simulink model "SF003A_Dampg"  (R2013b)
settings: Solver=FixedStepDiscrete  SolverMode=SingleTasking  StartTime=0.0  StopTime=1  FixedStep=.002  RelTol=1e-3
values from neighbouring files (symbols this model uses):
  ARCHGLBPRM_2MILLISEC_SEC_F32 = DataDict.Constant    [SF003A_Dampg_DataDict.m]
  DampgHydBasCoeff1 = DataDict.Calibration    [SF003A_Dampg_DataDict.m]
  DampgHydBasCoeff2 = DataDict.Calibration    [SF003A_Dampg_DataDict.m]
  DampgHydBasCoeff3 = DataDict.Calibration    [SF003A_Dampg_DataDict.m]
  DampgHydBasCoeff4 = DataDict.Calibration    [SF003A_Dampg_DataDict.m]
  DampgHydOutpLim = DataDict.Calibration    [SF003A_Dampg_DataDict.m]
  DampgQuad13Mplr = DataDict.Calibration    [SF003A_Dampg_DataDict.m]
  DampgQuad24Mplr = DataDict.Calibration    [SF003A_Dampg_DataDict.m]
  DampgQuadHwTqBacklsh = DataDict.Calibration    [SF003A_Dampg_DataDict.m]
  DampgQuadMotVelBacklsh = DataDict.Calibration    [SF003A_Dampg_DataDict.m]
  FLTINJ_DAMPG_DAMPGCMDBAS = DataDict.Constant    [SF003A_Dampg_DataDict.m]
libraries: FloatToFixd x9, Fil x8, FixdToFloat x8, LnrIntrpn x7, NxtrAbslt x5, NxtrSign x3, NxtrLim x3, simulink x1, NxtrMax x1, BilnrIntrpnMplX x1
(part 2 of 2)

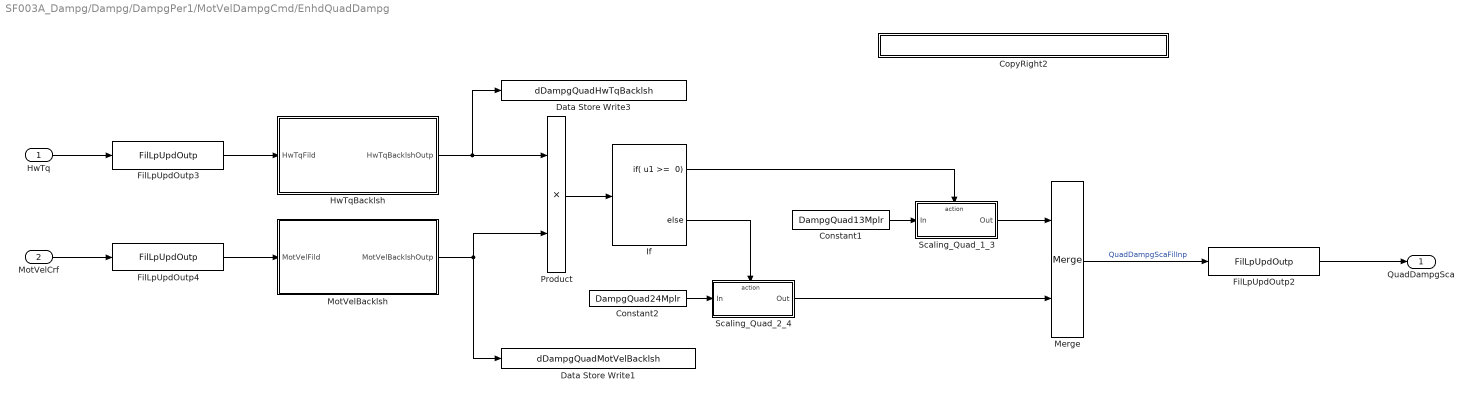
== system SF003A_Dampg/Dampg/DampgPer1/MotVelDampgCmd/EnhdQuadDampg  ==
  HwTq : Inport
  MotVelCrf : Inport  Port=2
  Constant1 : Constant  RequirementInfo={'linktype_rmi_doors' '0000a525 (/E-STEER Core/SubSystem Specifications/Application Functions/SF003A Damping)' '#SF003A_113' 'true' 'REQ: SF003A_113' '' } %GIDa_5b902024_3e8c_4494_84c3_91dcbfea766a  Value=DampgQuad13Mplr  OutDataTypeStr=single
  Constant2 : Constant  RequirementInfo={'linktype_rmi_doors' '0000a525 (/E-STEER Core/SubSystem Specifications/Application Functions/SF003A Damping)' '#SF003A_114' 'true' 'REQ: SF003A_114' '' } %GIDa_587e475f_d2d7_438f_8480_63dc4e95efa6  Value=DampgQuad24Mplr  OutDataTypeStr=single
  CopyRight2 : Subsystem  Description=|  mask(Copyright Information){none=on}
      | Copyright info block.                                               
      |                                                                     
      | Place copyright information at the top of every subsystem in design.
      mask prompts: none "No parameters"
      mask help: Place copyright information at the top of every subsystem in design.
      mask Display:
      | NxtrConf = 'Nexteer Confidential';
      | 
      | sys = bdroot; %handle for the current model ("system")
      | first = get_param(sys,'Created');
      | if(isempty(first))
      |     first = datestr(now,'yyyy');
      | else
      |     first = first(end-3:end);  %year is last four digits
      | end
      | 
      | last = get_param(sys,'LastModifiedDate');
      | if isempty(last)
      |     last = datestr(now,'yyyy');
      | else
      |     last = last(end-3:end);
      | end
      | 
      | if strcmp(first,last)
      |     fprintf('%s -- Copyright %s Nexteer',NxtrConf,first)
      | else
      |     fprintf('%s -- %s%s- %s Nexteer',NxtrConf,char(169),first,last)
      | end
  Data Store Write1 : DataStoreWrite  DataStoreName=dDampgQuadMotVelBacklsh
  Data Store Write3 : DataStoreWrite  DataStoreName=dDampgQuadHwTqBacklsh
  FilLpUpdOutp2 : Fil/FilLpUpdOutp  RequirementInfo={'linktype_rmi_doors' '0000a525 (/E-STEER Core/SubSystem Specifications/Application Functions/SF003A Damping)' '#SF003A_115' 'true' 'REQ: SF003A_115' '' } %GIDa_3cce034f_6843_47ba_883e_e9472d6bea51  StVar=QuadDampgScaLpFil
      settings: AttributesFormatString=StVar: %<StVar>
  FilLpUpdOutp3 : Fil/FilLpUpdOutp  RequirementInfo={'linktype_rmi_doors' '0000a525 (/E-STEER Core/SubSystem Specifications/Application Functions/SF003A Damping)' '#SF003A_135' 'true' 'REQ: SF003A_135' '' } %GIDa_4951c7ec_0e7d_4afa_9064_51627a057340  StVar=QuadDampgHwTqLpFil
      settings: AttributesFormatString=StVar: %<StVar>
  FilLpUpdOutp4 : Fil/FilLpUpdOutp  RequirementInfo={'linktype_rmi_doors' '0000a525 (/E-STEER Core/SubSystem Specifications/Application Functions/SF003A Damping)' '#SF003A_137' 'true' 'REQ: SF003A_137' '' } %GIDa_73f2fc1e_0696_4bfb_b3f7_ed9952c3095a  StVar=QuadDampgMotVelLpFil
      settings: AttributesFormatString=StVar: %<StVar>
  HwTqBacklsh : Subsystem  RequirementInfo={'linktype_rmi_doors' '0000a525 (/E-STEER Core/SubSystem Specifications/Application Functions/SF003A Damping)' '#SF003A_136' 'true' 'REQ: SF003A_136' '' } %GIDa_bd470be9_d6d9_40e9_857a_c378f7458848
  If : If  RequirementInfo={'linktype_rmi_doors' '0000a525 (/E-STEER Core/SubSystem Specifications/Application Functions/SF003A Damping)' '#SF003A_113' 'true' 'REQ: SF003A_113' '' ; 'linktype_rmi_doors' '0000a525 (/E-STEER Core/SubSystem Specifications/Application Functions/SF003A Damping)' '#SF003A_114' 'true' 'REQ: SF003A_114' '' } %GIDa_cfe1943d_8645_4c6c_ae36_bf006afd8732  IfExpression="u1 >=  0"
  Merge : Merge
  MotVelBacklsh : Subsystem  RequirementInfo={'linktype_rmi_doors' '0000a525 (/E-STEER Core/SubSystem Specifications/Application Functions/SF003A Damping)' '#SF003A_138' 'true' 'REQ: SF003A_138' '' } %GIDa_e894bb2d_e794_4ed4_a57e_9441dd65fceb
  Product : Product  RndMeth=Zero
  Scaling_Quad_1_3 : Subsystem  RequirementInfo={'linktype_rmi_doors' '0000a525 (/E-STEER Core/SubSystem Specifications/Application Functions/SF003A Damping)' '#SF003A_113' 'true' 'REQ: SF003A_113' '' } %GIDa_485cad3f_31a8_4856_95a7_16cb3f5dc668  TreatAsAtomicUnit=on
  Scaling_Quad_2_4 : Subsystem  RequirementInfo={'linktype_rmi_doors' '0000a525 (/E-STEER Core/SubSystem Specifications/Application Functions/SF003A Damping)' '#SF003A_114' 'true' 'REQ: SF003A_114' '' } %GIDa_b28b5c6d_494b_445a_b5ee_da8ce8308b9a  TreatAsAtomicUnit=on
  QuadDampgSca : Outport
  wires:
  MotVelCrf/1 -> FilLpUpdOutp4/1
  HwTq/1 -> FilLpUpdOutp3/1
  MotVelBacklsh/1(MotVelBacklshOutp) -> Data Store Write1/1, Product/2
  Product/1 -> If/1
  If/1 -> Scaling_Quad_1_3/Action
  If/2 -> Scaling_Quad_2_4/Action
  Scaling_Quad_1_3/1(Out) -> Merge/1
  Merge/1 -> FilLpUpdOutp2/1  "QuadDampgScaFilInp"
  FilLpUpdOutp2/1 -> QuadDampgSca/1
  Constant1/1 -> Scaling_Quad_1_3/1(In)
  Constant2/1 -> Scaling_Quad_2_4/1(In)
  Scaling_Quad_2_4/1(Out) -> Merge/2
  FilLpUpdOutp4/1 -> MotVelBacklsh/1(MotVelFild)
  HwTqBacklsh/1(HwTqBacklshOutp) -> Data Store Write3/1, Product/1
  FilLpUpdOutp3/1 -> HwTqBacklsh/1(HwTqFild)

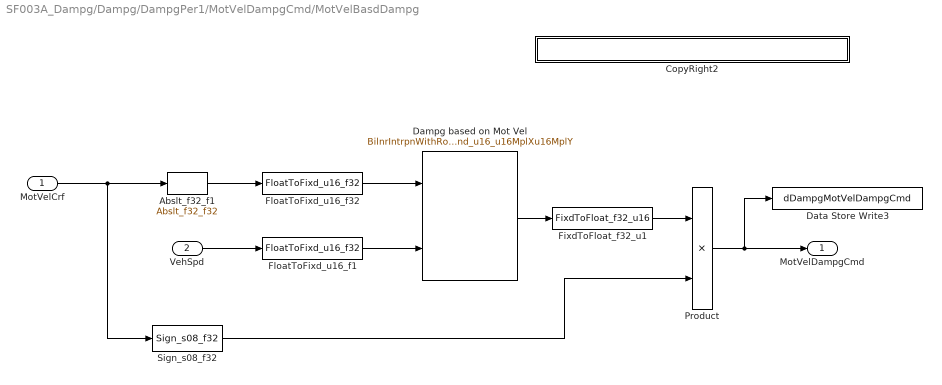
== system SF003A_Dampg/Dampg/DampgPer1/MotVelDampgCmd/MotVelBasdDampg ==
  MotVelCrf : Inport
  VehSpd : Inport  Port=2
  Abslt_f32_f1 : NxtrAbslt/Abslt_f32_f32  SFunctionSpec=single y1 = Abslt_f32_f32(single u1)
      settings: AttributesFormatString=%<Name>
  CopyRight2 : Subsystem  Description=|  mask(Copyright Information){none=on}
      | Copyright info block.                                               
      |                                                                     
      | Place copyright information at the top of every subsystem in design.
      mask prompts: none "No parameters"
      mask help: Place copyright information at the top of every subsystem in design.
      mask Display:
      | NxtrConf = 'Nexteer Confidential';
      | 
      | sys = bdroot; %handle for the current model ("system")
      | first = get_param(sys,'Created');
      | if(isempty(first))
      |     first = datestr(now,'yyyy');
      | else
      |     first = first(end-3:end);  %year is last four digits
      | end
      | 
      | last = get_param(sys,'LastModifiedDate');
      | if isempty(last)
      |     last = datestr(now,'yyyy');
      | else
      |     last = last(end-3:end);
      | end
      | 
      | if strcmp(first,last)
      |     fprintf('%s -- Copyright %s Nexteer',NxtrConf,first)
      | else
      |     fprintf('%s -- %s%s- %s Nexteer',NxtrConf,char(169),first,last)
      | end
  Dampg based on Mot Vel : BilnrIntrpnMplX/BilnrIntrpnWithRound_u16_u16MplXu16MplY  RequirementInfo={'linktype_rmi_doors' '0000a525 (/E-STEER Core/SubSystem Specifications/Application Functions/SF003A Damping)' '#SF003A_116' 'true' 'REQ: SF003A_116' '' } %GIDa_ea730993_70af_440c_875a_3fc7509d9afc  MplXTbl=DampgMotVelX  MplYTbl=DampgMotVelY  BilnrSelnTbl=SysGlbPrmVehSpdBilnrSeln
      settings: AttributesFormatString=Bilnr ( u16MplX , u16MplY )
  Data Store Write3 : DataStoreWrite  DataStoreName=dDampgMotVelDampgCmd
  FixdToFloat_f32_u1 : FixdToFloat/FixdToFloat_f32_u16  RequirementInfo={'linktype_rmi_doors' '0000a525 (/E-STEER Core/SubSystem Specifications/Application Functions/SF003A Damping)' '#SF003A_116' 'true' 'REQ: SF003A_116' '' } %GIDa_a554a576_bc87_4218_8687_13e7c762261c  Param1=11
  FloatToFixd_u16_f1 : FloatToFixd/FloatToFixd_u16_f32  RequirementInfo={'linktype_rmi_doors' '0000a525 (/E-STEER Core/SubSystem Specifications/Application Functions/SF003A Damping)' '#SF003A_116' 'true' 'REQ: SF003A_116' '' } %GIDa_3b87165c_8634_4461_8108_249e587b1972  Param1=7
  FloatToFixd_u16_f32 : FloatToFixd/FloatToFixd_u16_f32  RequirementInfo={'linktype_rmi_doors' '0000a525 (/E-STEER Core/SubSystem Specifications/Application Functions/SF003A Damping)' '#SF003A_116' 'true' 'REQ: SF003A_116' '' } %GIDa_acfe93e2_2d64_4d5a_9389_bd02cf1ec0ad  Param1=4
  Product : Product  RequirementInfo={'linktype_rmi_doors' '0000a525 (/E-STEER Core/SubSystem Specifications/Application Functions/SF003A Damping)' '#SF003A_117' 'true' 'REQ: SF003A_117' '' } %GIDa_9410abb1_72c1_467c_b827_70e405450db0  RndMeth=Zero
  Sign_s08_f32 : NxtrSign/Sign_s08_f32  RequirementInfo={'linktype_rmi_doors' '0000a525 (/E-STEER Core/SubSystem Specifications/Application Functions/SF003A Damping)' '#SF003A_117' 'true' 'REQ: SF003A_117' '' } %GIDa_8898375e_9dcb_4cf2_ba9b_f98fb975f09b  SFunctionSpec=int8 y1 = Sign_s08_f32(single u1)
  MotVelDampgCmd : Outport
  wires:
  Sign_s08_f32/1 -> Product/2
  MotVelCrf/1 -> Abslt_f32_f1/1, Sign_s08_f32/1
  FloatToFixd_u16_f32/1 -> Dampg based on Mot Vel/1
  FloatToFixd_u16_f1/1 -> Dampg based on Mot Vel/2
  Dampg based on Mot Vel/1 -> FixdToFloat_f32_u1/1
  Abslt_f32_f1/1 -> FloatToFixd_u16_f32/1
  VehSpd/1 -> FloatToFixd_u16_f1/1
  Product/1 -> Data Store Write3/1, MotVelDampgCmd/1
  FixdToFloat_f32_u1/1 -> Product/1

== system SF003A_Dampg/Dampg/DampgPer1/CmdDiChk/DmpgCmdChk/CopyRight2 ==

== system SF003A_Dampg/Dampg/DampgPer1/CmdDiChk/Zero_Command/CopyRight2 ==

== system SF003A_Dampg/Dampg/DampgPer1/MotVelDampgCmd/EnhdQuadDampg /CopyRight2 ==

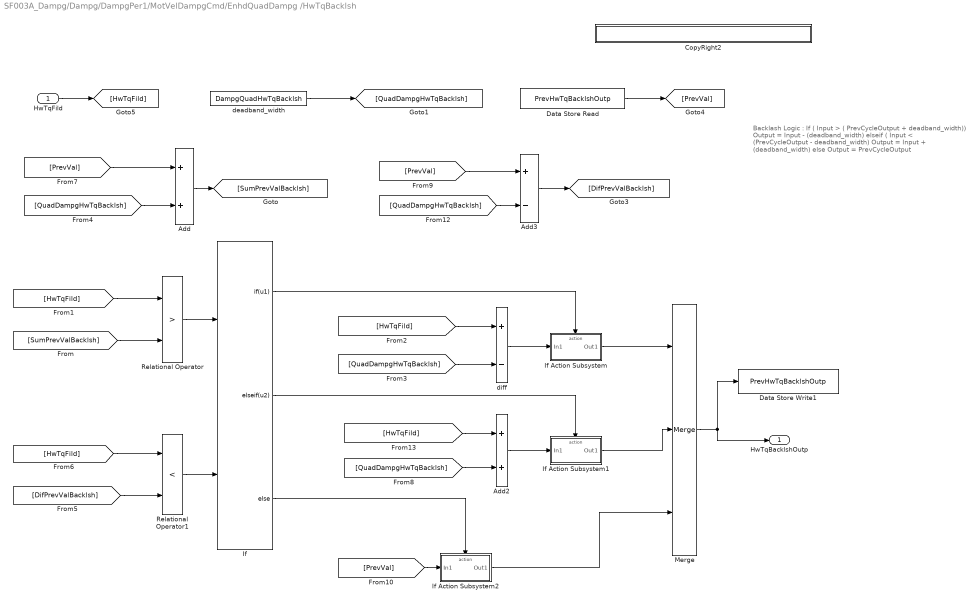
== system SF003A_Dampg/Dampg/DampgPer1/MotVelDampgCmd/EnhdQuadDampg /HwTqBacklsh ==
  note: Backlash Logic :
      | If ( Input > ( PrevCycleOutput + deadband_width))
      | 	Output = Input - (deadband_width)
      | elseif ( Input < (PrevCycleOutput - deadband_width)
      | 	Output = Input + (deadband_width)
      | else
      | 	Output = PrevCycleOutput
  HwTqFild : Inport
  Add : Sum
  Add2 : Sum
  Add3 : Sum  Inputs=+-
  CopyRight2 : Subsystem  Description=|  mask(Copyright Information){none=on}
      | Copyright info block.                                               
      |                                                                     
      | Place copyright information at the top of every subsystem in design.
      mask prompts: none "No parameters"
      mask help: Place copyright information at the top of every subsystem in design.
      mask Display:
      | NxtrConf = 'Nexteer Confidential';
      | 
      | sys = bdroot; %handle for the current model ("system")
      | first = get_param(sys,'Created');
      | if(isempty(first))
      |     first = datestr(now,'yyyy');
      | else
      |     first = first(end-3:end);  %year is last four digits
      | end
      | 
      | last = get_param(sys,'LastModifiedDate');
      | if isempty(last)
      |     last = datestr(now,'yyyy');
      | else
      |     last = last(end-3:end);
      | end
      | 
      | if strcmp(first,last)
      |     fprintf('%s -- Copyright %s Nexteer',NxtrConf,first)
      | else
      |     fprintf('%s -- %s%s- %s Nexteer',NxtrConf,char(169),first,last)
      | end
  Data Store Read : DataStoreRead  DataStoreName=PrevHwTqBacklshOutp
  Data Store Write1 : DataStoreWrite  DataStoreName=PrevHwTqBacklshOutp
  If : If  NumInputs=2  IfExpression=u1  ElseIfExpressions=u2
  If Action Subsystem : Subsystem  TreatAsAtomicUnit=on
  If Action Subsystem1 : Subsystem  TreatAsAtomicUnit=on
  If Action Subsystem2 : Subsystem  TreatAsAtomicUnit=on
  Merge : Merge  Inputs=3
  Relational Operator : RelationalOperator  Operator=>  OutDataTypeStr=boolean
  Relational Operator1 : RelationalOperator  Operator=<  OutDataTypeStr=boolean
  deadband_width : Constant  Value=DampgQuadHwTqBacklsh  OutDataTypeStr=single
  diff : Sum  Inputs=+-
  HwTqBacklshOutp : Outport
  wires:
  Relational Operator/1 -> If/1
  [SumPrevValBacklsh] -> Relational Operator/2
  [HwTqFild] -> Relational Operator/1
  diff/1 -> If Action Subsystem/1(In1)
  [HwTqFild] -> diff/1
  [QuadDampgHwTqBacklsh] -> diff/2
  If/1 -> If Action Subsystem/Action
  [HwTqFild] -> Relational Operator1/1
  [DifPrevValBacklsh] -> Relational Operator1/2
  Relational Operator1/1 -> If/2
  [HwTqFild] -> Add2/1
  [QuadDampgHwTqBacklsh] -> Add2/2
  Add2/1 -> If Action Subsystem1/1(In1)
  If/2 -> If Action Subsystem1/Action
  [PrevVal] -> If Action Subsystem2/1(In1)
  If/3 -> If Action Subsystem2/Action
  If Action Subsystem1/1(Out1) -> Merge/2
  If Action Subsystem2/1(Out1) -> Merge/3
  If Action Subsystem/1(Out1) -> Merge/1
  Merge/1 -> HwTqBacklshOutp/1, Data Store Write1/1
  deadband_width/1 -> [QuadDampgHwTqBacklsh]
  Add/1 -> [SumPrevValBacklsh]
  [PrevVal] -> Add/1
  [QuadDampgHwTqBacklsh] -> Add/2
  Add3/1 -> [DifPrevValBacklsh]
  [PrevVal] -> Add3/1
  [QuadDampgHwTqBacklsh] -> Add3/2
  Data Store Read/1 -> [PrevVal]
  HwTqFild/1 -> [HwTqFild]

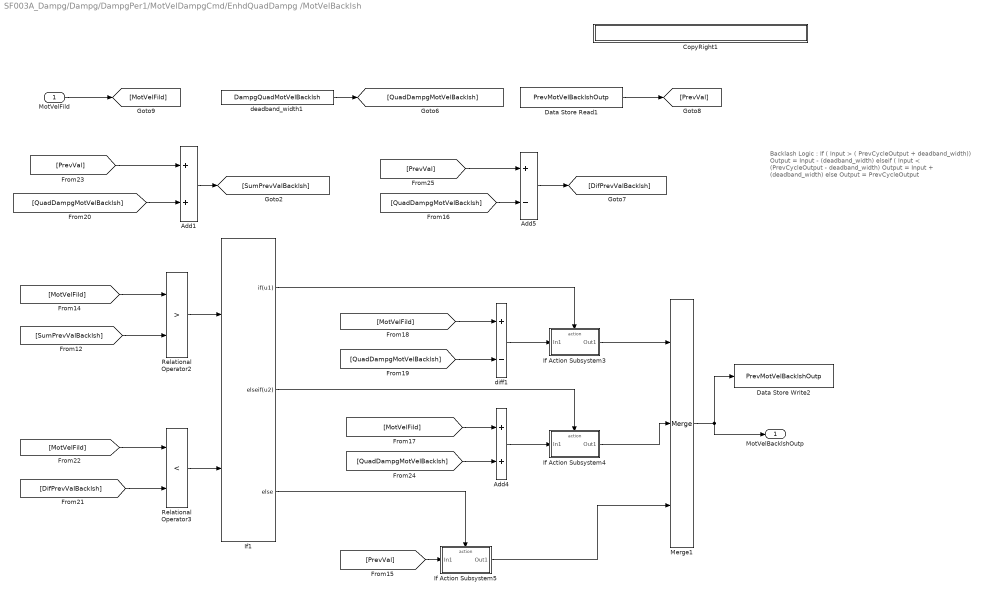
== system SF003A_Dampg/Dampg/DampgPer1/MotVelDampgCmd/EnhdQuadDampg /MotVelBacklsh ==
  note: Backlash Logic :
      | If ( Input > ( PrevCycleOutput + deadband_width))
      | 	Output = Input - (deadband_width)
      | elseif ( Input < (PrevCycleOutput - deadband_width)
      | 	Output = Input + (deadband_width)
      | else
      | 	Output = PrevCycleOutput
  MotVelFild : Inport
  Add1 : Sum
  Add4 : Sum
  Add5 : Sum  Inputs=+-
  CopyRight1 : Subsystem  Description=|  mask(Copyright Information){none=on}
      | Copyright info block.                                               
      |                                                                     
      | Place copyright information at the top of every subsystem in design.
      mask prompts: none "No parameters"
      mask help: Place copyright information at the top of every subsystem in design.
      mask Display:
      | NxtrConf = 'Nexteer Confidential';
      | 
      | sys = bdroot; %handle for the current model ("system")
      | first = get_param(sys,'Created');
      | if(isempty(first))
      |     first = datestr(now,'yyyy');
      | else
      |     first = first(end-3:end);  %year is last four digits
      | end
      | 
      | last = get_param(sys,'LastModifiedDate');
      | if isempty(last)
      |     last = datestr(now,'yyyy');
      | else
      |     last = last(end-3:end);
      | end
      | 
      | if strcmp(first,last)
      |     fprintf('%s -- Copyright %s Nexteer',NxtrConf,first)
      | else
      |     fprintf('%s -- %s%s- %s Nexteer',NxtrConf,char(169),first,last)
      | end
  Data Store Read1 : DataStoreRead  DataStoreName=PrevMotVelBacklshOutp
  Data Store Write2 : DataStoreWrite  DataStoreName=PrevMotVelBacklshOutp
  If Action Subsystem3 : Subsystem  TreatAsAtomicUnit=on
  If Action Subsystem4 : Subsystem  TreatAsAtomicUnit=on
  If Action Subsystem5 : Subsystem  TreatAsAtomicUnit=on
  If1 : If  NumInputs=2  IfExpression=u1  ElseIfExpressions=u2
  Merge1 : Merge  Inputs=3
  Relational Operator2 : RelationalOperator  Operator=>  OutDataTypeStr=boolean
  Relational Operator3 : RelationalOperator  Operator=<  OutDataTypeStr=boolean
  deadband_width1 : Constant  Value=DampgQuadMotVelBacklsh  OutDataTypeStr=single
  diff1 : Sum  Inputs=+-
  MotVelBacklshOutp : Outport
  wires:
  Relational Operator2/1 -> If1/1
  [SumPrevValBacklsh] -> Relational Operator2/2
  [MotVelFild] -> Relational Operator2/1
  diff1/1 -> If Action Subsystem3/1(In1)
  [MotVelFild] -> diff1/1
  [QuadDampgMotVelBacklsh] -> diff1/2
  If1/1 -> If Action Subsystem3/Action
  [MotVelFild] -> Relational Operator3/1
  [DifPrevValBacklsh] -> Relational Operator3/2
  Relational Operator3/1 -> If1/2
  [MotVelFild] -> Add4/1
  [QuadDampgMotVelBacklsh] -> Add4/2
  Add4/1 -> If Action Subsystem4/1(In1)
  If1/2 -> If Action Subsystem4/Action
  [PrevVal] -> If Action Subsystem5/1(In1)
  If1/3 -> If Action Subsystem5/Action
  If Action Subsystem4/1(Out1) -> Merge1/2
  If Action Subsystem5/1(Out1) -> Merge1/3
  If Action Subsystem3/1(Out1) -> Merge1/1
  Merge1/1 -> MotVelBacklshOutp/1, Data Store Write2/1
  deadband_width1/1 -> [QuadDampgMotVelBacklsh]
  Add1/1 -> [SumPrevValBacklsh]
  [PrevVal] -> Add1/1
  [QuadDampgMotVelBacklsh] -> Add1/2
  Add5/1 -> [DifPrevValBacklsh]
  [PrevVal] -> Add5/1
  [QuadDampgMotVelBacklsh] -> Add5/2
  Data Store Read1/1 -> [PrevVal]
  MotVelFild/1 -> [MotVelFild]

== system SF003A_Dampg/Dampg/DampgPer1/MotVelDampgCmd/EnhdQuadDampg /Scaling_Quad_1_3 ==
  In : Inport
  Action Port : ActionPort  ActionType=then
  CopyRight2 : Subsystem  Description=|  mask(Copyright Information){none=on}
      | Copyright info block.                                               
      |                                                                     
      | Place copyright information at the top of every subsystem in design.
      mask prompts: none "No parameters"
      mask help: Place copyright information at the top of every subsystem in design.
      mask Display:
      | NxtrConf = 'Nexteer Confidential';
      | 
      | sys = bdroot; %handle for the current model ("system")
      | first = get_param(sys,'Created');
      | if(isempty(first))
      |     first = datestr(now,'yyyy');
      | else
      |     first = first(end-3:end);  %year is last four digits
      | end
      | 
      | last = get_param(sys,'LastModifiedDate');
      | if isempty(last)
      |     last = datestr(now,'yyyy');
      | else
      |     last = last(end-3:end);
      | end
      | 
      | if strcmp(first,last)
      |     fprintf('%s -- Copyright %s Nexteer',NxtrConf,first)
      | else
      |     fprintf('%s -- %s%s- %s Nexteer',NxtrConf,char(169),first,last)
      | end
  Out : Outport
  wires:
  In/1 -> Out/1

== system SF003A_Dampg/Dampg/DampgPer1/MotVelDampgCmd/EnhdQuadDampg /Scaling_Quad_2_4 ==
  In : Inport
  Action Port : ActionPort  ActionType=else
  CopyRight2 : Subsystem  Description=|  mask(Copyright Information){none=on}
      | Copyright info block.                                               
      |                                                                     
      | Place copyright information at the top of every subsystem in design.
      mask prompts: none "No parameters"
      mask help: Place copyright information at the top of every subsystem in design.
      mask Display:
      | NxtrConf = 'Nexteer Confidential';
      | 
      | sys = bdroot; %handle for the current model ("system")
      | first = get_param(sys,'Created');
      | if(isempty(first))
      |     first = datestr(now,'yyyy');
      | else
      |     first = first(end-3:end);  %year is last four digits
      | end
      | 
      | last = get_param(sys,'LastModifiedDate');
      | if isempty(last)
      |     last = datestr(now,'yyyy');
      | else
      |     last = last(end-3:end);
      | end
      | 
      | if strcmp(first,last)
      |     fprintf('%s -- Copyright %s Nexteer',NxtrConf,first)
      | else
      |     fprintf('%s -- %s%s- %s Nexteer',NxtrConf,char(169),first,last)
      | end
  Out : Outport
  wires:
  In/1 -> Out/1

== system SF003A_Dampg/Dampg/DampgPer1/MotVelDampgCmd/MotVelBasdDampg/CopyRight2 ==

== system SF003A_Dampg/Dampg/DampgPer1/MotVelDampgCmd/EnhdQuadDampg /HwTqBacklsh/CopyRight2 ==

== system SF003A_Dampg/Dampg/DampgPer1/MotVelDampgCmd/EnhdQuadDampg /HwTqBacklsh/If Action Subsystem ==
  In1 : Inport
  Action Port : ActionPort  ActionType=then
  CopyRight2 : Subsystem  Description=|  mask(Copyright Information){none=on}
      | Copyright info block.                                               
      |                                                                     
      | Place copyright information at the top of every subsystem in design.
      mask prompts: none "No parameters"
      mask help: Place copyright information at the top of every subsystem in design.
      mask Display:
      | NxtrConf = 'Nexteer Confidential';
      | 
      | sys = bdroot; %handle for the current model ("system")
      | first = get_param(sys,'Created');
      | if(isempty(first))
      |     first = datestr(now,'yyyy');
      | else
      |     first = first(end-3:end);  %year is last four digits
      | end
      | 
      | last = get_param(sys,'LastModifiedDate');
      | if isempty(last)
      |     last = datestr(now,'yyyy');
      | else
      |     last = last(end-3:end);
      | end
      | 
      | if strcmp(first,last)
      |     fprintf('%s -- Copyright %s Nexteer',NxtrConf,first)
      | else
      |     fprintf('%s -- %s%s- %s Nexteer',NxtrConf,char(169),first,last)
      | end
  Out1 : Outport
  wires:
  In1/1 -> Out1/1

== system SF003A_Dampg/Dampg/DampgPer1/MotVelDampgCmd/EnhdQuadDampg /HwTqBacklsh/If Action Subsystem1 ==
  In1 : Inport
  Action Port : ActionPort  ActionType=elseif
  CopyRight2 : Subsystem  Description=|  mask(Copyright Information){none=on}
      | Copyright info block.                                               
      |                                                                     
      | Place copyright information at the top of every subsystem in design.
      mask prompts: none "No parameters"
      mask help: Place copyright information at the top of every subsystem in design.
      mask Display:
      | NxtrConf = 'Nexteer Confidential';
      | 
      | sys = bdroot; %handle for the current model ("system")
      | first = get_param(sys,'Created');
      | if(isempty(first))
      |     first = datestr(now,'yyyy');
      | else
      |     first = first(end-3:end);  %year is last four digits
      | end
      | 
      | last = get_param(sys,'LastModifiedDate');
      | if isempty(last)
      |     last = datestr(now,'yyyy');
      | else
      |     last = last(end-3:end);
      | end
      | 
      | if strcmp(first,last)
      |     fprintf('%s -- Copyright %s Nexteer',NxtrConf,first)
      | else
      |     fprintf('%s -- %s%s- %s Nexteer',NxtrConf,char(169),first,last)
      | end
  Out1 : Outport
  wires:
  In1/1 -> Out1/1

== system SF003A_Dampg/Dampg/DampgPer1/MotVelDampgCmd/EnhdQuadDampg /HwTqBacklsh/If Action Subsystem2 ==
  In1 : Inport
  Action Port : ActionPort  ActionType=else
  CopyRight2 : Subsystem  Description=|  mask(Copyright Information){none=on}
      | Copyright info block.                                               
      |                                                                     
      | Place copyright information at the top of every subsystem in design.
      mask prompts: none "No parameters"
      mask help: Place copyright information at the top of every subsystem in design.
      mask Display:
      | NxtrConf = 'Nexteer Confidential';
      | 
      | sys = bdroot; %handle for the current model ("system")
      | first = get_param(sys,'Created');
      | if(isempty(first))
      |     first = datestr(now,'yyyy');
      | else
      |     first = first(end-3:end);  %year is last four digits
      | end
      | 
      | last = get_param(sys,'LastModifiedDate');
      | if isempty(last)
      |     last = datestr(now,'yyyy');
      | else
      |     last = last(end-3:end);
      | end
      | 
      | if strcmp(first,last)
      |     fprintf('%s -- Copyright %s Nexteer',NxtrConf,first)
      | else
      |     fprintf('%s -- %s%s- %s Nexteer',NxtrConf,char(169),first,last)
      | end
  Out1 : Outport
  wires:
  In1/1 -> Out1/1

== system SF003A_Dampg/Dampg/DampgPer1/MotVelDampgCmd/EnhdQuadDampg /MotVelBacklsh/CopyRight1 ==

== system SF003A_Dampg/Dampg/DampgPer1/MotVelDampgCmd/EnhdQuadDampg /MotVelBacklsh/If Action Subsystem3 ==
  In1 : Inport
  Action Port : ActionPort  ActionType=then
  CopyRight2 : Subsystem  Description=|  mask(Copyright Information){none=on}
      | Copyright info block.                                               
      |                                                                     
      | Place copyright information at the top of every subsystem in design.
      mask prompts: none "No parameters"
      mask help: Place copyright information at the top of every subsystem in design.
      mask Display:
      | NxtrConf = 'Nexteer Confidential';
      | 
      | sys = bdroot; %handle for the current model ("system")
      | first = get_param(sys,'Created');
      | if(isempty(first))
      |     first = datestr(now,'yyyy');
      | else
      |     first = first(end-3:end);  %year is last four digits
      | end
      | 
      | last = get_param(sys,'LastModifiedDate');
      | if isempty(last)
      |     last = datestr(now,'yyyy');
      | else
      |     last = last(end-3:end);
      | end
      | 
      | if strcmp(first,last)
      |     fprintf('%s -- Copyright %s Nexteer',NxtrConf,first)
      | else
      |     fprintf('%s -- %s%s- %s Nexteer',NxtrConf,char(169),first,last)
      | end
  Out1 : Outport
  wires:
  In1/1 -> Out1/1

== system SF003A_Dampg/Dampg/DampgPer1/MotVelDampgCmd/EnhdQuadDampg /MotVelBacklsh/If Action Subsystem4 ==
  In1 : Inport
  Action Port : ActionPort  ActionType=elseif
  CopyRight2 : Subsystem  Description=|  mask(Copyright Information){none=on}
      | Copyright info block.                                               
      |                                                                     
      | Place copyright information at the top of every subsystem in design.
      mask prompts: none "No parameters"
      mask help: Place copyright information at the top of every subsystem in design.
      mask Display:
      | NxtrConf = 'Nexteer Confidential';
      | 
      | sys = bdroot; %handle for the current model ("system")
      | first = get_param(sys,'Created');
      | if(isempty(first))
      |     first = datestr(now,'yyyy');
      | else
      |     first = first(end-3:end);  %year is last four digits
      | end
      | 
      | last = get_param(sys,'LastModifiedDate');
      | if isempty(last)
      |     last = datestr(now,'yyyy');
      | else
      |     last = last(end-3:end);
      | end
      | 
      | if strcmp(first,last)
      |     fprintf('%s -- Copyright %s Nexteer',NxtrConf,first)
      | else
      |     fprintf('%s -- %s%s- %s Nexteer',NxtrConf,char(169),first,last)
      | end
  Out1 : Outport
  wires:
  In1/1 -> Out1/1

== system SF003A_Dampg/Dampg/DampgPer1/MotVelDampgCmd/EnhdQuadDampg /MotVelBacklsh/If Action Subsystem5 ==
  In1 : Inport
  Action Port : ActionPort  ActionType=else
  CopyRight2 : Subsystem  Description=|  mask(Copyright Information){none=on}
      | Copyright info block.                                               
      |                                                                     
      | Place copyright information at the top of every subsystem in design.
      mask prompts: none "No parameters"
      mask help: Place copyright information at the top of every subsystem in design.
      mask Display:
      | NxtrConf = 'Nexteer Confidential';
      | 
      | sys = bdroot; %handle for the current model ("system")
      | first = get_param(sys,'Created');
      | if(isempty(first))
      |     first = datestr(now,'yyyy');
      | else
      |     first = first(end-3:end);  %year is last four digits
      | end
      | 
      | last = get_param(sys,'LastModifiedDate');
      | if isempty(last)
      |     last = datestr(now,'yyyy');
      | else
      |     last = last(end-3:end);
      | end
      | 
      | if strcmp(first,last)
      |     fprintf('%s -- Copyright %s Nexteer',NxtrConf,first)
      | else
      |     fprintf('%s -- %s%s- %s Nexteer',NxtrConf,char(169),first,last)
      | end
  Out1 : Outport
  wires:
  In1/1 -> Out1/1

== system SF003A_Dampg/Dampg/DampgPer1/MotVelDampgCmd/EnhdQuadDampg /Scaling_Quad_1_3/CopyRight2 ==

== system SF003A_Dampg/Dampg/DampgPer1/MotVelDampgCmd/EnhdQuadDampg /Scaling_Quad_2_4/CopyRight2 ==

== system SF003A_Dampg/Dampg/DampgPer1/MotVelDampgCmd/EnhdQuadDampg /HwTqBacklsh/If Action Subsystem/CopyRight2 ==

== system SF003A_Dampg/Dampg/DampgPer1/MotVelDampgCmd/EnhdQuadDampg /HwTqBacklsh/If Action Subsystem1/CopyRight2 ==

== system SF003A_Dampg/Dampg/DampgPer1/MotVelDampgCmd/EnhdQuadDampg /HwTqBacklsh/If Action Subsystem2/CopyRight2 ==

== system SF003A_Dampg/Dampg/DampgPer1/MotVelDampgCmd/EnhdQuadDampg /MotVelBacklsh/If Action Subsystem3/CopyRight2 ==

== system SF003A_Dampg/Dampg/DampgPer1/MotVelDampgCmd/EnhdQuadDampg /MotVelBacklsh/If Action Subsystem4/CopyRight2 ==

== system SF003A_Dampg/Dampg/DampgPer1/MotVelDampgCmd/EnhdQuadDampg /MotVelBacklsh/If Action Subsystem5/CopyRight2 ==
